simulink model "simulinkCart_ROS_GAZEBO-pratica5"  (R2023b)
settings: Solver=ode4  StartTime=0.0  StopTime=100  FixedStep=0.001  RelTol=1e-3
undefined symbols (not defined in the file or in its folder): angular, linear
libraries: simulink x6, ros2lib x4, Controllers x1
settings Model: Creator=calebe  LastModifiedBy=calebe
settings OptimizationCC: EnhancedBackFolding=on  PassReuseOutputArgsAs=Individual arguments  ZeroExternalMemoryAtStartup=off  ZeroInternalMemoryAtStartup=off  MaxStackSize=64  OptimizeBlockOrder=speed  DifferentSizesBufferReuse=on  OptimizationCustomize=off  EfficientTunableParamExpr=on
settings DebuggingCC: ParameterTunabilityLossMsg=error
settings HardwareCC: ProdBitPerLong=64  ProdHWDeviceType=Intel->x86-64 (Linux 64)
settings SFSimCC: MATLABDynamicMemAlloc=off
settings RTWCC: Description=Embedded Coder  SystemTargetFile=ert.tlc  HardwareBoard=Robot Operating System 2 (ROS 2)  TLCOptions="-aInlineSetEventsForThisBaseRateFcn=TLC_FALSE -aSuppressMultiTaskScheduler=TLC_FALSE  -aRateBasedStepFcn=0"  TemplateMakefile=ert_default_tmf  Toolchain=Colcon Tools  TargetLang=C++
settings CodeAppCC: ForceParamTrailComments=on  IgnoreCustomStorageClasses=off  OperatorAnnotations=on  SimulinkDataObjDesc=on  SFDataObjDesc=on  InsertBlockDesc=on
settings ERTTargetCC: CodeInterfacePackaging=C++ class  RootIOFormat=Structure reference

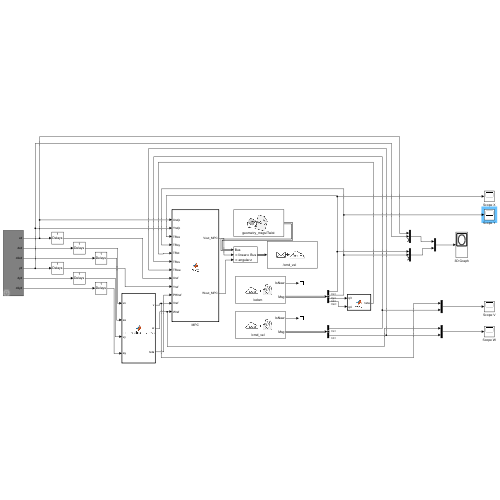
[thumbnail: Simulink's stored preview of the top-level diagram]
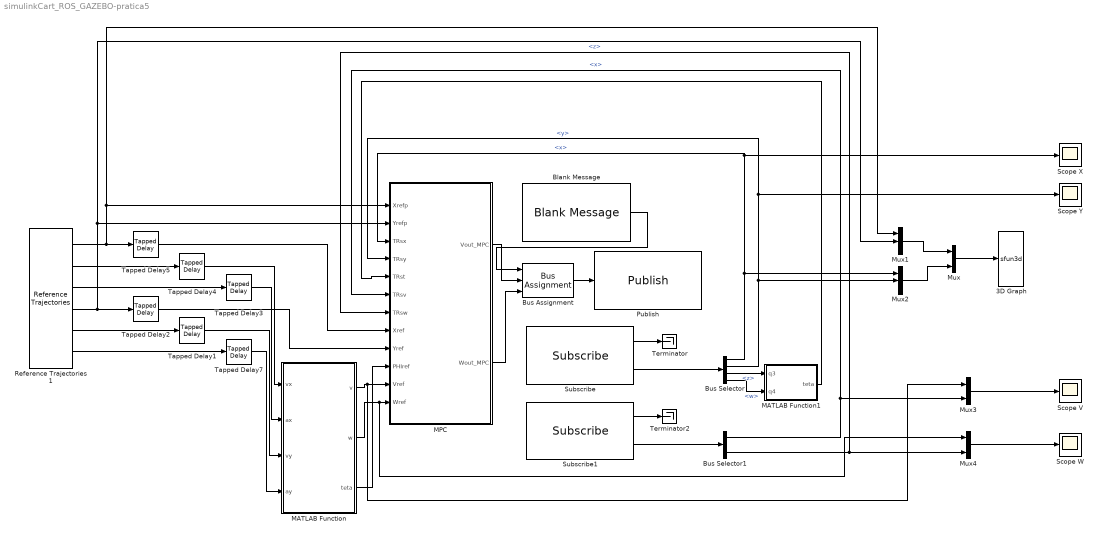
== system simulinkCart_ROS_GAZEBO-pratica5 ==
  3D Graph : S-Function  LoadFcn=if exist('sfun3d','file'), sfun3d([],[],[],'LoadBlock'); end  FunctionName=sfun3d  Parameters=ax,T,np,cp,gd,ls,mk,mx,hd,tb  SFunctionDeploymentMode=off  EnableBusSupport=off  mask(3D Graph){np=2, ax=[-3 3 -3 3 -3 3], mx=1e4, T=0.04, cp=[0 0 1], gd=on, hd=off, tb=off, ls=-, mk=none}
      mask prompts: np "Number of moving points (lines)"; ax "Range: [xmin xmax  ymin ymax zmin zmax]"; mx "Max number of points in each line"; T "Sampling Time"; cp "Camera position (use [0 0 1] for 2D XY view)"; gd "Grid (on|off)"; hd "HeadMarkers (on|off)"; tb "Toolbar (on|off)"; ls "LineStyle"; mk "LineMarker"
      mask help:
      | This block plots the position of several points in the XYZ space. The input contains the coordinates of all the points (x1,y1,z1,x2,y2,z2,...).
      | The number of moving points (lines), the XYZ ranges, sampling time, camera position, and grid (among other things) can be set as mask parameters.
      settings: CopyFcn=if exist('sfun3d','file'), sfun3d([],[],[],'CopyBlock'); end  DeleteFcn=if exist('sfun3d','file'), sfun3d([],[],[],'DeleteBlock'); end  NameChangeFcn=if exist('sfun3d','file'), sfun3d([],[],[],'NameChange'); end
      mask Help:
      | This block plots the position of several points in the XYZ space. The input contains the coordinates of all the points (x1,y1,z1,x2,y2,z2,...).
      | The number of moving points (lines), the XYZ ranges, sampling time, camera position, and grid (among other things) can be set as mask parameters.
      mask TypeOptions ls: - | -- | : | -. | none
      mask TypeOptions mk: none | . | + | o | * | x | square | diamond | v | ^ | > | < | pentagram | hexagram
      mask Display: plot([.05 .95 .95 .05 .05],[.45 .45 .95 .95 .45], 0.5+cos(0:0.1:2*pi)*0.3,0.7+sin(0:0.1:2*pi)*0.2)
  Blank Message : ros2lib/Blank Message  messageClass=Message  entityType=geometry_msgs/Twist  messageType=geometry_msgs/Twist  SampleTime=inf
  Bus Assignment : BusAssignment  AssignedSignals=linear.x,angular.z
  Bus Selector : BusSelector  OutputSignals=pose.pose.position.x,pose.pose.position.y,pose.pose.orientation.z,pose.pose.orientation.w
  Bus Selector1 : BusSelector  OutputSignals=linear.x,angular.z
  MATLAB Function : MATLAB Function  TreatAsAtomicUnit=on
  MATLAB Function1 : MATLAB Function  TreatAsAtomicUnit=on
  MPC : MATLAB Function  TreatAsAtomicUnit=on
  Mux : Mux  Inputs=2
  Mux1 : Mux  Inputs=3
  Mux2 : Mux  Inputs=3
  Mux3 : Mux  Inputs=2
  Mux4 : Mux  Inputs=2
  Publish : ros2lib/Publish  topicSource=Select from ROS network  topic=/cmd_vel  messageType=geometry_msgs/Twist  QOSHistory=Keep last  QOSDepth=1  QOSReliability=Reliable  QOSDurability=Volatile
  Reference Trajectories1 : Controllers/Reference Trajectories  trajectory_type=2  wf=0.1  raio_ref_1=1  delta_raio=0  t_delta_raio=60  xd=[1, -1.5]
  Scope V : Scope
  Scope W : Scope
  Scope X : Scope
  Scope Y : Scope
  Subscribe : ros2lib/Subscribe  topicSource=Select from ROS network  topic=/odom  messageType=nav_msgs/Odometry  sampleTime=-1  QOSHistory=Keep last  QOSDepth=1  QOSReliability=Reliable  QOSDurability=Volatile
  Subscribe1 : ros2lib/Subscribe  topicSource=Select from ROS network  topic=/cmd_vel  messageType=geometry_msgs/Twist  sampleTime=-1  QOSHistory=Keep last  QOSDepth=1  QOSReliability=Reliable  QOSDurability=Volatile
  Tapped Delay{1..5,7} (6 alike) : simulink/Discrete/Tapped Delay  vinit=0.0  samptime=-1  NumDelays=1  DelayOrder=Oldest  includeCurrent=off
  Terminator : Terminator
  Terminator2 : Terminator
  wires:
  Mux1/1 -> Mux/1
  Mux2/1 -> Mux/2
  Mux/1 -> 3D Graph/1
  Reference Trajectories1/2 -> Tapped Delay4/1
  Reference Trajectories1/3 -> Tapped Delay3/1
  Reference Trajectories1/5 -> Tapped Delay1/1
  Reference Trajectories1/6 -> Tapped Delay7/1
  Tapped Delay5/1 -> MPC/8(Xref)
  Tapped Delay2/1 -> MPC/9(Yref)
  Tapped Delay4/1 -> MATLAB Function/1(vx)
  Tapped Delay3/1 -> MATLAB Function/2(ax)
  Tapped Delay1/1 -> MATLAB Function/3(vy)
  Tapped Delay7/1 -> MATLAB Function/4(ay)
  MATLAB Function/3(teta) -> MPC/10(PHIref)
  MATLAB Function/2(w) -> Mux4/1, MPC/12(Wref)
  Blank Message/1 -> Bus Assignment/1
  Bus Assignment/1 -> Publish/1
  MPC/1(Vout_MPC) -> Bus Assignment/2
  MPC/2(Wout_MPC) -> Bus Assignment/3
  Subscribe/1 -> Terminator/1
  Subscribe/2 -> Bus Selector/1
  Subscribe1/1 -> Terminator2/1
  Subscribe1/2 -> Bus Selector1/1
  Bus Selector/1 -> Mux2/1, MPC/3(TRsx), Scope X/1  "<x>"
  Bus Selector/2 -> Mux2/2, MPC/4(TRsy), Scope Y/1  "<y>"
  Bus Selector1/1 -> Mux3/2, MPC/6(TRsv)  "<x>"
  Bus Selector/3 -> MATLAB Function1/1(q3)  "<z>"
  Bus Selector/4 -> MATLAB Function1/2(q4)  "<w>"
  Bus Selector1/2 -> Mux4/2, MPC/7(TRsw)  "<z>"
  MATLAB Function1/1(teta) -> MPC/5(TRst)
  Mux3/1 -> Scope V/1
  Mux4/1 -> Scope W/1
  MATLAB Function/1(v) -> Mux3/1, MPC/11(Vref)
  Reference Trajectories1/1 -> MPC/1(Xrefp), Mux1/1, Tapped Delay5/1
  Reference Trajectories1/4 -> Mux1/2, MPC/2(Yrefp), Tapped Delay2/1

== matlab function simulinkCart_ROS_GAZEBO-pratica5/MATLAB Function1 ==
  data: q3 input; teta output; q4 input
function teta = fcn2(q3, q4)
%#codegen
teta = 2*atan2(q3, q4);

== matlab function simulinkCart_ROS_GAZEBO-pratica5/MPC ==
  data: Xrefp input; Vout_MPC output; Yrefp input; TRsx input; TRsy input; TRst input; TRsv input; TRsw input; Xref input; Yref input; PHIref input; Vref input; Wref input; Wout_MPC output
function [Vout_MPC,Wout_MPC]=MPC(Xrefp, Yrefp, TRsx, TRsy, TRst,TRsv,TRsw, Xref, Yref, PHIref, Vref, Wref)
%#codegen
% Este é o código completo do "cérebro" MPC, baseado no Passo 20 da Prática 4.
% Esta versão está LIMPA, sem os erros de citação.

% --- Passo 20.a: Configuração dos Parâmetros do Controlador ---
Vmax = 0.4;
d = 0.23;
N1 = 1;
N2 = 10;
Nu = 2;
L1 = 10;
L2 = 2000;
L3 = 0.05;
eta = 0.1;
Imax = 15;
I = 0;
Delta = 0.1;

% --- Passo 20.b: Configuração dos Parâmetros do Otimizador ---
alpha = 0.015;

% --- Passo 20.c: Inicialização dos vetores do Otimizador ---
Jsteps = zeros(8, 1);
Jgrad = zeros(4, 1);
Jgrad_prev = zeros(4, 1);

% --- Passo 20.d: Inicializando modelo do preditor ---
Ubest = zeros(2, 2);
Uref = zeros(2, 2);
Uaux = zeros(2, 2);
SimRob = struct('x', 0, 'y', 0, 'teta', 0, 'v', 0, 'w', 0); 

% --- Passo 20.e: INICIALIZAÇÃO DAS VARIÁVEIS DO CONTROLADOR ---

% 20.e.i: Inicialização da Saída de Controle Desejada
Uref(1,1) = Vref;
Uref(2,1) = Wref;
Uref(1,2) = Vref;
Uref(2,2) = Wref;

% 20.e.ii: Cálculo da Trajetória de Referência
% (Esta função 'calcRefTraj' deve estar no seu .zip)
[tPX,tPY,tPTeta] = calcRefTraj(0.01, TRsx, TRsy, TRst, Xref, Yref, PHIref, Vref, Wref, N2, Xrefp, Yrefp);

% 20.e.iii: Atualiza Modelo do Preditor
SimRob.x = TRsx;
SimRob.y = TRsy;
SimRob.teta = TRst;
SimRob.v = TRsv;
SimRob.w = TRsw;

% --- Passo 20.f: INÍCIO DO LOOP DE CONTROLE ---

% 20.f.i: Satura as Velocidades
% (Esta função 'scaleForSaturation' deve estar no seu .zip)
Uref = scaleForSaturation(Uref, d, Nu, Vmax);

% 20.f.ii: Calcula o Valor Inicial da Função Custo J
Jatual = COST_FUNCTION(SimRob.x, SimRob.y, SimRob.teta, SimRob.v, SimRob.w, Uref, tPX, tPY, tPTeta, N1, N2, Nu, L1, L2, L3);
Jbest = Jatual;
Ubest = Uref;

% 20.f.iii: INÍCIO DO LOOP DE OTIMIZAÇÃO
I = 0; % Zerando o contador I
while (I < Imax && Jatual > eta)
    
    % 20.f.iv: Calcula os Passos (Usteps)
    Usteps = calcUsteps(Uref, Nu, Delta);
    
    % 20.f.v: Cálculo de todos os J para o horizonte
    for k = 0:1:Nu-1
        for j = 1:1:4
            % 1. Atribui velocidades para cada passo
            for m = 0:1:Nu-1
                if m == k
                    Uaux(1,m+1) = Usteps(1,(j+4*k));
                    Uaux(2,m+1) = Usteps(2,(j+4*k));
                else
                    Uaux(1,m+1) = Uref(1,m+1);
                    Uaux(2,m+1) = Uref(2,m+1);
                end
            end
            
            % 2. Reinicia a posição inicial
            SimRob.x = TRsx;
            SimRob.y = TRsy;
            SimRob.teta = TRst;
            SimRob.v = TRsv;
            SimRob.w = TRsw;
            
            % 3. Satura novamente
            % (Esta função 'scaleForSaturation' deve estar no seu .zip)
            Uaux = scaleForSaturation(Uaux, d, Nu, Vmax);
            
            % 4. Calcula o J da iteração
            J = COST_FUNCTION(SimRob.x, SimRob.y, SimRob.teta, SimRob.v, SimRob.w, Uaux, tPX, tPY, tPTeta, N1, N2, Nu, L1, L2, L3);
            Jsteps(j+4*k, 1) = J;
        end
    end
    
    % 20.f.vi: Calcula o Gradiente de J
    for h = 0:1:Nu-1
        Jgrad_prev(2*h+1,1) = Jgrad(2*h+1,1);
        Jgrad(2*h+1,1) = Jsteps(4*h+1,1) - Jsteps(4*h+2,1);
        
        Jgrad_prev(2*h+2,1) = Jgrad(2*h+2,1);
        Jgrad(2*h+2,1) = Jsteps(4*h+3,1) - Jsteps(4*h+4,1);
    end
    
    % 20.f.vii: Cálculo do Gradiente Conjugado
    di = [0 0];
    x1 = di;
    for z = 0:1:Nu-1
        di(1) = Jgrad(2*z+1,1);
        di(2) = Jgrad(2*z+2,1);
        
        x1(1) = (Uref(1,z+1) - alpha*di(1));
        x1(2) = (Uref(2,z+1) - alpha*di(2));
        
        Jgrad_prev(2*z+1,1) = Jgrad(2*z+1,1);
        Jgrad(2*z+1,1) = Jsteps(4*z+1,1) - Jsteps(4*z+2,1);
        Jgrad_prev(2*z+2,1) = Jgrad(2*z+2,1);
        Jgrad(2*z+2,1) = Jsteps(4*z+3,1) - Jsteps(4*z+4,1);
        
        beta = 0;
        if ((Jgrad(2*z+1,1) >= eta) || (Jgrad(2*z+2,1) >= eta))
            t1 = (Jgrad(2*z+1,1) - Jgrad_prev(2*z+1,1));
            t2 = (Jgrad(2*z+2,1) - Jgrad_prev(2*z+2,1));
            a1 = (Jgrad(2*z+1,1) * t1);
            a2 = (Jgrad(2*z+2,1) * t2);
            b1 = (Jgrad_prev(2*z+1,1) * Jgrad_prev(2*z+1,1));
            b2 = (Jgrad_prev(2*z+2,1) * Jgrad_prev(2*z+2,1));
            if (b1+b2) ~= 0 % Evitar divisão por zero
                beta = ((a1+a2)/(b1+b2));
            end
        end
        
        Uref(1,z+1) = x1(1) + alpha*(-Jgrad(2*z+1,1) + beta*Jgrad_prev(2*z+1,1));
        Uref(2,z+1) = x1(2) + alpha*(-Jgrad(2*z+2,1) + beta*Jgrad_prev(2*z+2,1));
    end
    
    % 20.f.viii: Reinicia Posição
    SimRob.x = TRsx;
    SimRob.y = TRsy;
    SimRob.teta = TRst;
    SimRob.v = TRsv;
    SimRob.w = TRsw;
    
    % 20.f.ix: Satura Velocidade
    % (Esta função 'scaleForSaturation' deve estar no seu .zip)
    Uref = scaleForSaturation(Uref, d, Nu, Vmax);
    
    % 20.f.x: Recalcula J Atual
    Jatual = COST_FUNCTION(SimRob.x, SimRob.y, SimRob.teta, SimRob.v, SimRob.w, Uref, tPX, tPY, tPTeta, N1, N2, Nu, L1, L2, L3);
    
    % 20.f.xi: Testa se J é melhor
    if Jatual < Jbest
        Jbest = Jatual;
        Ubest = Uref;
    end
    
    I = I + 1;
end % Fim do loop 'while'

% --- Passo 20.g: SAÍDA DO CONTROLADOR ---
Vout_MPC = Ubest(1, 1);
Wout_MPC = Ubest(2, 1);


% =================================================================
% --- FUNÇÕES LOCAIS (NESTED FUNCTIONS) ---
% =l================================================================

% --- Função COST_FUNCTION (Baseada na descrição 20.f.ii.1-5) ---
function J = COST_FUNCTION(x, y, teta, v, w, U, tPX, tPY, tPTeta, N1, N2, Nu, L1, L2, L3)
    
    % 1. Zera variáveis de soma
    sumX = 0;
    sumY = 0;
    sumT = 0;
    sum_dU = 0;
    
    % Prepara a simulação do robô
    SimRob.x = x;
    SimRob.y = y;
    SimRob.teta = teta;
    
    % 2. Define tempo discreto
    t = 0.01;
    
    % 3. Inicia laço de N1 a N2
    for i = N1:N2
        
        % a. Atribui velocidades
        current_U_index = i;
        if i > Nu
            current_U_index = Nu;
        end
        v_sim = U(1, current_U_index);
        w_sim = U(2, current_U_index);
        
        % b. Inicia laço de simulação interna (4 passos de 0.01s = 0.04s)
        for j = 1:4
            % i. Realiza simulação (slide 44 da aula_3.pdf)
            SimRob.teta = SimRob.teta + w_sim * t;
            SimRob.x = SimRob.x + v_sim * cos(SimRob.teta) * t;
            SimRob.y = SimRob.y + v_sim * sin(SimRob.teta) * t;
        end
        
        % c. Realiza somatório da função custo
        ex = SimRob.x - tPX(i);
        ey = SimRob.y - tPY(i);
        eT = DiffAngle(SimRob.teta, tPTeta(i));
        
        sumX = sumX + ex^2;
        sumY = sumY + ey^2;
        sumT = sumT + eT^2;
    end
    
    % 4. Somatório da variação de velocidades
    for i = 1:Nu-1
        sum_dU = sum_dU + (U(1,i+1) - U(1,i))^2 + (U(2,i+1) - U(2,i))^2;
    end
    
    % 5. Custo Total
    J = L1*(sumX + sumY) + L2*sumT + L3*sum_dU;
end


% --- Função Auxiliar: Diff Angle ---
function[ang] = DiffAngle(a1,a2)
    ang = a1-a2;
    if ang < 0
        ang = -((-ang/(2*pi)) - floor((-ang/(2*pi))) * 2*pi);
    end
    if ang < -pi
        ang = ang + 2*pi;
    else
        ang = ((ang/(2*pi)) - floor((ang/(2*pi)))) * (2*pi);
    end
    if ang > pi
        ang = ang - 2*pi;
    end
end

% --- Função Auxiliar: calcUsteps ---
function[dU] = calcUsteps(U, Nu, delta)
    dU = zeros(2,(Nu*4));
    for i=0:1:Nu-1
        dU(1,1+4*i) = U(1,i+1) + delta;
        dU(2,1+4*i) = U(2,i+1);
        
        dU(1,2+4*i) = U(1,i+1) - delta;
        dU(2,2+4*i) = U(2,i+1);
        
        dU(1,3+4*i) = U(1,i+1);
        dU(2,3+4*i) = U(2,i+1) + delta;
        
        dU(1,4+4*i) = U(1,i+1);
        dU(2,4+4*i) = U(2,i+1) - delta;
    end
end


end % <--- ESTE É O 'END' FINAL QUE FECHA A FUNÇÃO 'MPC'

== matlab function simulinkCart_ROS_GAZEBO-pratica5/MATLAB Function ==
  data: vx input; v output; ax input; vy input; ay input; w output; teta output
function [v, w, teta] = cinematica_inversa(vx, ax, vy, ay)
%#codegen
% Este bloco implementa a Cinemática Inversa do Passo 17
% Entradas: [vx, ax, vy, ay] (velocidades e acelerações do Mundo)
% Saídas: [v, w, teta] (velocidades e ângulo do Robô)

% Fórmula para 'v' (Velocidade Linear)
% v = sqrt(vx^2 + vy^2)
% (aula_3.pdf, slide 44-45)
v = sqrt(vx^2 + vy^2);

% Fórmula para 'teta' (Ângulo do Robô)
% teta = atan2(vy, vx)
% (aula_3.pdf, slide 44-45)
teta = atan2(vy, vx);

% Fórmula para 'w' (Velocidade Angular)
% w = (ay*vx - ax*vy) / (vx^2 + vy^2)
% (aula_3.pdf, slide 44-45)
if (v < 0.001)
    % Evita divisão por zero se a velocidade for muito baixa
    w = 0;
else
    w = (ay*vx - ax*vy) / (vx^2 + vy^2);
end

end
